simulink model "Leg_4DOF_HGO_noise"  (R2017a)
settings: Solver=FixedStepAuto  StartTime=0.0  StopTime=15  FixedStep=simulation_step  MaxStep=1e-2  RelTol=1e-3  EnableMultiTasking=on
values from neighbouring files (symbols this model uses):
  Amp = [ 1 ; pi/2*ones(3,1) ]    [Copy_of_Init_4DOF.m]
  Ar = [zeros(4) eye(4); zeros(4) zeros(4)]    [Copy_of_Init_HGO_v2.m]    (also in Init_HGO.m; Init_HGO_v1.m; Init_HGO_zoh_v2.m)
  beta = 10    [Copy_of_Init_4DOF.m]
  BodyContact = [ 4 4 ]    [Copy_of_Init_4DOF.m]
  BodyContactPositions = [ contact_point_h, contact_point_t ]    [Copy_of_Init_4DOF.m]
  Br = [zeros(4); eye(4)]    [Copy_of_Init_HGO_v2.m]    (also in Init_HGO.m; Init_HGO_v1.m; Init_HGO_zoh_v2.m)
  Cr = [eye(4) zeros(4)]    [Copy_of_Init_HGO_v2.m]    (also in Init_HGO.m; Init_HGO_v1.m; Init_HGO_zoh_v2.m)
  dqInit = [ 0 0 0 0 ]'    [Copy_of_Init_4DOF.m]
  G = g*ez    [Copy_of_Init_4DOF.m]
  G_ctrl = g*ez    [Copy_of_Init_4DOF.m]
  h = [ ez -ey -ey -ey ]    [Copy_of_Init_4DOF.m]
  h_ctrl = [ ez -ey -ey -ey ]    [Copy_of_Init_4DOF.m]
  Hmu = [eye(4)/Mu zeros(4); zeros(4) eye(4)/Mu^2]    [Copy_of_Init_HGO_v2.m]    (also in Init_HGO.m; Init_HGO_v1.m; Init_HGO_zoh_v2.m)
  Inertia = [ I_base I_hip I_thigh I_shin I_foot ]    [Copy_of_Init_4DOF.m]
  Inertia_ctrl = [ I_base I_hip I_thigh I_shin I_foot ]    [Copy_of_Init_4DOF.m]
  joint_type = [ 1 0 0 0 ]    [Copy_of_Init_4DOF.m]
  k_b = 10    [Copy_of_Init_4DOF.m]
  Kd = kd*eye(n)    [Copy_of_Init_4DOF.m]
  Ki = ki*eye(n)    [Copy_of_Init_4DOF.m]
  Kp = kp*eye(n)    [Copy_of_Init_4DOF.m]
  L = [ l_base_hip l_hip_thigh l_thigh_shin l_shin_foot ]    [Copy_of_Init_4DOF.m]
  L_ctrl = [ l_base_hip l_hip_thigh l_thigh_shin l_shin_foot ]    [Copy_of_Init_4DOF.m]
  L_hgo = [2*eye(4);6*eye(4)]    [Copy_of_Init_HGO_v2.m]    (also in Init_HGO.m = [eye(4);2*eye(4)]; Init_HGO_v1.m = [eye(4);2*eye(4)]; Init_HGO_zoh_v2.m)
  Mass = [ mass_base mass_hip mass_thigh mass_shin mass_foot ]    [Copy_of_Init_4DOF.m]
  Mass_ctrl = [ mass_base mass_hip mass_thigh mass_shin mass_foot ]    [Copy_of_Init_4DOF.m]
  Mu = 1e-3    (= 0.001)    [Copy_of_Init_HGO_v2.m]    (also in Init_HGO.m = 0.005; Init_HGO_v1.m; Init_HGO_zoh_v2.m = 1e-05)
  offset = zeros(n,1)    [Copy_of_Init_4DOF.m]
  qInit = [ 0 pi/2 -pi/2 0 ]'    [Copy_of_Init_4DOF.m]
  R = [ r_base r_hip r_thigh r_shin r_foot ]    [Copy_of_Init_4DOF.m]
  R_ctrl = [ r_base r_hip r_thigh r_shin r_foot ]    [Copy_of_Init_4DOF.m]
  s_z = 2    [Copy_of_Init_4DOF.m]
  w = [ 0   ; 0.5*pi*ones(3,1) ]    [Copy_of_Init_4DOF.m]
undefined symbols (not defined in the file or in its folder): filter_pole, Fstate0, magnitude, simulation_step, step_period
libraries: commchan3 x1
Description:
  | ------ 2018-03-01
  | ------V2
  | Versão com realimentacao de estados estimados (HGO), apresenta
  | resposta lenta devido ao pico no inicio das estimativas.
  | Ainda nao possui medidor de SNR.
settings Model: Creator=Ultron  LastModifiedBy=ignacio
settings DataIOCC: LimitDataPoints=on  SaveFormat=Array
settings OptimizationCC: LifeSpan=inf
settings DebuggingCC: SFUnexpectedBacktrackingDiag=warning  SFNoUnconditionalDefaultTransitionDiag=warning  SFExecutionAtInitializationDiag=none
settings HardwareCC: ProdBitPerPointer=32  ProdBitPerSizeT=32  ProdBitPerPtrDiffT=32  ProdLargestAtomicFloat=None  ProdIntDivRoundTo=Undefined  ProdEndianess=Unspecified  ProdWordSize=32  ProdHWDeviceType=32-bit Generic
settings ModelReferenceCC: PropagateSignalLabelsOutOfModel=off
settings GRTTargetCC: TargetLangStandard=C89/C90 (ANSI)  GeneratePreprocessorConditionals=Disable all
settings ConfigComp: CovMetricSettings=dw  CovHtmlReporting=on  CovSaveCumulativeToWorkspaceVar=on  CovSaveSingleToWorkspaceVar=on  CovExternalEMLEnable=off

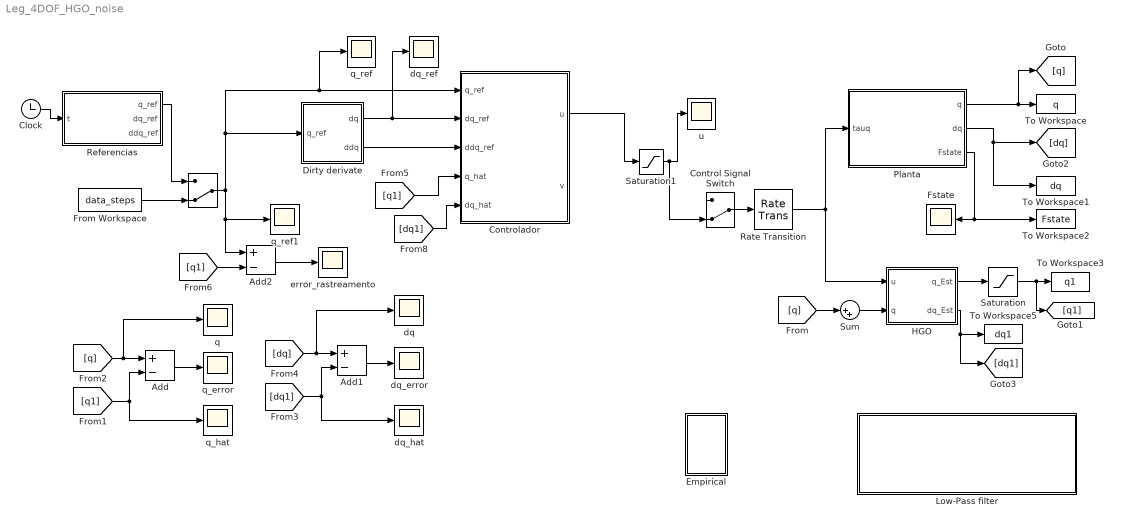
== system Leg_4DOF_HGO_noise ==
  " " : ManualSwitch  CurrentSetting=0
  Add : Sum  Inputs=+-
  Add1 : Sum  Inputs=+-
  Add2 : Sum  Inputs=+-
  Clock : Clock
  Control Signal Switch : ManualSwitch  CurrentSetting=0
  Controlador : Subsystem
  Dirty derivate : Subsystem
  Empirical : Subsystem
  From Workspace : FromWorkspace  VariableName=data_steps  SampleTime=0
  Fstate : Scope
  HGO : Subsystem
  Low-Pass filter : Subsystem
  Planta : Subsystem
  Rate Transition : RateTransition  OutPortSampleTime=simulation_step
  Referencias : MATLAB Function  TreatAsAtomicUnit=on
  Saturation : Saturate  UpperLimit=6*pi  LowerLimit=-6*pi
  Saturation1 : Saturate  UpperLimit=500  LowerLimit=-500
  Sum : Sum  Inputs=|++
  To Workspace : ToWorkspace  VariableName=q  SaveFormat=Timeseries  SampleTime=-1
  To Workspace1 : ToWorkspace  VariableName=dq  SaveFormat=Timeseries  SampleTime=-1
  To Workspace2 : ToWorkspace  VariableName=Fstate  SaveFormat=Timeseries  SampleTime=-1
  To Workspace3 : ToWorkspace  VariableName=q1  SaveFormat=Timeseries  SampleTime=-1
  To Workspace5 : ToWorkspace  VariableName=dq1  SaveFormat=Timeseries  SampleTime=-1
  dq : Scope
  dq_error : Scope
  dq_hat : Scope
  dq_ref : Scope
  error_rastreamento : Scope
  q : Scope
  q_error : Scope
  q_hat : Scope
  q_ref : Scope
  q_ref1 : Scope
  u : Scope
  wires:
  HGO/2(dq_Est) -> To Workspace5/1, [dq1]
  Sum/1 -> HGO/2(q)
  [q] -> Sum/1
  Saturation/1 -> [q1], To Workspace3/1
  [q1] -> q_hat/1, Add/2
  Clock/1 -> Referencias/1(t)
  [dq] -> dq/1, Add1/1
  Dirty derivate/2(ddq) -> Controlador/3(ddq_ref)
  Rate Transition/1 -> HGO/1(u), Planta/1(tauq)
  Dirty derivate/1(dq) -> dq_ref/1, Controlador/2(dq_ref)
  [dq1] -> dq_hat/1, Add1/2
  [q1] -> Controlador/4(q_hat)
  Planta/3(Fstate) -> Fstate/1, To Workspace2/1
  Referencias/1(q_ref) -> " "/1
  Add1/1 -> dq_error/1
  From Workspace/1 -> " "/2
  " "/1 -> Add2/1, q_ref1/1, Controlador/1(q_ref), q_ref/1, Dirty derivate/1(q_ref)
  HGO/1(q_Est) -> Saturation/1
  Planta/2(dq) -> To Workspace1/1, [dq]
  [dq1] -> Controlador/5(dq_hat)
  [q] -> q/1, Add/1
  Saturation1/1 -> Control Signal Switch/2, u/1
  Control Signal Switch/1 -> Rate Transition/1
  Controlador/1(u) -> Saturation1/1
  Add/1 -> q_error/1
  Planta/1(q) -> To Workspace/1, [q]
  [q1] -> Add2/2
  Add2/1 -> error_rastreamento/1

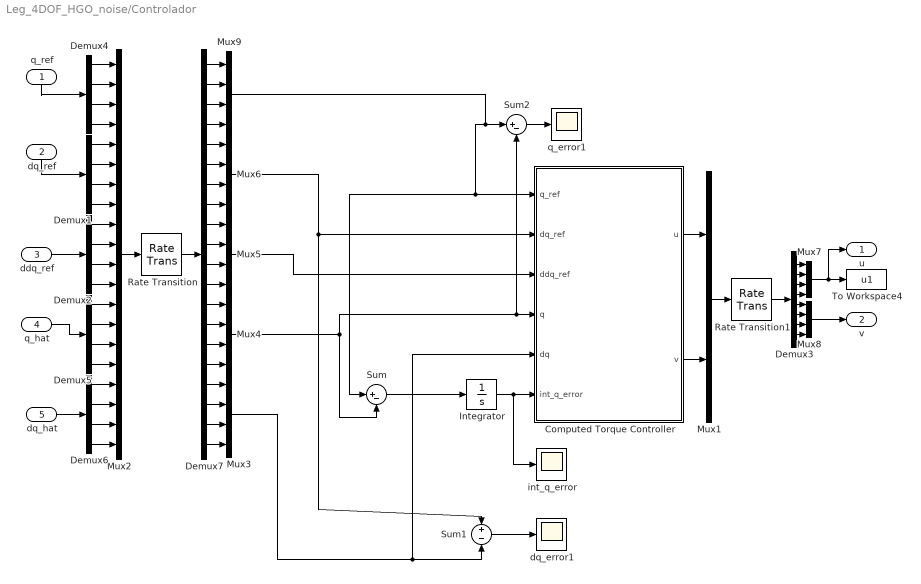
== system Leg_4DOF_HGO_noise/Controlador ==
  q_ref : Inport
  dq_ref : Inport  Port=2
  ddq_ref : Inport  Port=3
  q_hat : Inport  Port=4
  dq_hat : Inport  Port=5
  Computed Torque Controller : MATLAB Function  TreatAsAtomicUnit=on
  Demux{1..2,4..6} (5 alike) : Demux
  Demux3 : Demux  Outputs=8
  Demux7 : Demux  Outputs=20
  Integrator : Integrator  InitialCondition=zeros(4,1)
  Mux1 : Mux  Inputs=2
  Mux2 : Mux  Inputs=20
  Mux{3..9} (7 alike) : Mux
  Rate Transition : RateTransition  OutPortSampleTime=simulation_step
  Rate Transition1 : RateTransition  OutPortSampleTime=1e-3
  Sum : Sum  Inputs=|+-
  Sum1 : Sum  Inputs=+|-
  Sum2 : Sum  Inputs=|+-
  To Workspace4 : ToWorkspace  VariableName=u1  SaveFormat=Timeseries  SampleTime=-1
  dq_error1 : Scope
  int_q_error : Scope
  q_error1 : Scope
  u : Outport
  v : Outport  Port=2
  wires:
  Demux3/6 -> Mux8/2
  Demux6/3 -> Mux2/19
  Demux7/20 -> Mux3/4
  Mux3/1 -> Sum1/2, Computed Torque Controller/5(dq)
  dq_hat/1 -> Demux6/1
  Computed Torque Controller/1(u) -> Mux1/1
  Demux2/1 -> Mux2/9
  Demux1/3 -> Mux2/7
  Demux3/2 -> Mux7/2
  Sum1/1 -> dq_error1/1
  Demux6/2 -> Mux2/18
  q_ref/1 -> Demux4/1
  Demux5/4 -> Mux2/16
  Demux7/7 -> Mux6/3
  Demux7/16 -> Mux4/4
  Demux5/2 -> Mux2/14
  Demux7/3 -> Mux9/3
  Demux1/1 -> Mux2/5
  Demux6/1 -> Mux2/17
  Demux3/5 -> Mux8/1
  Mux6/1 -> Sum1/1, Computed Torque Controller/2(dq_ref)
  Demux3/4 -> Mux7/4
  q_hat/1 -> Demux5/1
  Demux7/5 -> Mux6/1
  Demux6/4 -> Mux2/20
  Demux3/3 -> Mux7/3
  Demux1/4 -> Mux2/8
  Mux9/1 -> Sum/1, Computed Torque Controller/1(q_ref), Sum2/1
  Mux8/1 -> v/1
  Mux4/1 -> Sum/2, Computed Torque Controller/4(q), Sum2/2
  Demux5/1 -> Mux2/13
  dq_ref/1 -> Demux1/1
  Demux2/3 -> Mux2/11
  Demux4/1 -> Mux2/1
  ddq_ref/1 -> Demux2/1
  Demux7/13 -> Mux4/1
  Demux3/7 -> Mux8/3
  Demux1/2 -> Mux2/6
  Demux2/4 -> Mux2/12
  Demux7/8 -> Mux6/4
  Demux7/6 -> Mux6/2
  Demux7/11 -> Mux5/3
  Demux7/9 -> Mux5/1
  Demux7/19 -> Mux3/3
  Demux7/1 -> Mux9/1
  Demux3/1 -> Mux7/1
  Sum2/1 -> q_error1/1
  Demux7/4 -> Mux9/4
  Demux7/14 -> Mux4/2
  Demux4/4 -> Mux2/4
  Demux7/12 -> Mux5/4
  Mux5/1 -> Computed Torque Controller/3(ddq_ref)
  Demux2/2 -> Mux2/10
  Demux7/2 -> Mux9/2
  Demux7/10 -> Mux5/2
  Integrator/1 -> int_q_error/1, Computed Torque Controller/6(int_q_error)
  Demux7/17 -> Mux3/1
  Demux7/18 -> Mux3/2
  Demux4/2 -> Mux2/2
  Sum/1 -> Integrator/1
  Computed Torque Controller/2(v) -> Mux1/2
  Demux3/8 -> Mux8/4
  Mux7/1 -> To Workspace4/1, u/1
  Demux4/3 -> Mux2/3
  Demux7/15 -> Mux4/3
  Demux5/3 -> Mux2/15
  Mux2/1 -> Rate Transition/1
  Rate Transition/1 -> Demux7/1
  Mux1/1 -> Rate Transition1/1
  Rate Transition1/1 -> Demux3/1

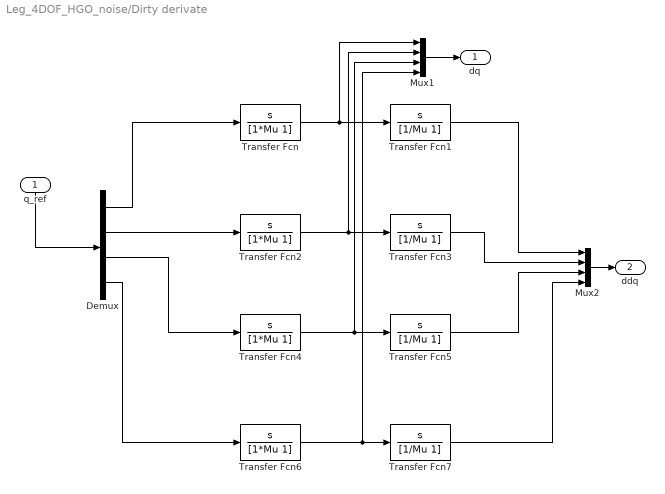
== system Leg_4DOF_HGO_noise/Dirty derivate ==
  q_ref : Inport
  Demux : Demux
  Mux1 : Mux
  Mux2 : Mux
  Transfer Fcn{,2,4,6} (4 alike) : TransferFcn  Numerator=[1 0]  Denominator=[1*Mu 1]
  Transfer Fcn{1,3,5,7} (4 alike) : TransferFcn  Numerator=[1 0]  Denominator=[1/Mu 1]
  dq : Outport
  ddq : Outport  Port=2
  wires:
  Transfer Fcn/1 -> Mux1/1, Transfer Fcn1/1
  q_ref/1 -> Demux/1
  Demux/1 -> Transfer Fcn/1
  Transfer Fcn6/1 -> Mux1/4, Transfer Fcn7/1
  Demux/2 -> Transfer Fcn2/1
  Demux/3 -> Transfer Fcn4/1
  Demux/4 -> Transfer Fcn6/1
  Mux1/1 -> dq/1
  Transfer Fcn4/1 -> Mux1/3, Transfer Fcn5/1
  Transfer Fcn2/1 -> Mux1/2, Transfer Fcn3/1
  Transfer Fcn1/1 -> Mux2/1
  Transfer Fcn3/1 -> Mux2/2
  Transfer Fcn5/1 -> Mux2/3
  Mux2/1 -> ddq/1
  Transfer Fcn7/1 -> Mux2/4

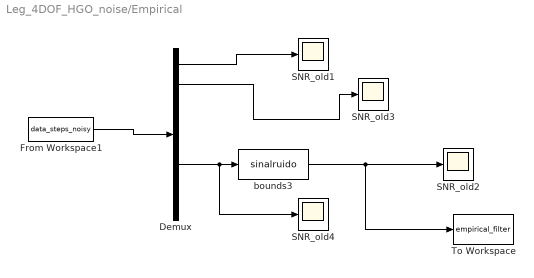
== system Leg_4DOF_HGO_noise/Empirical ==
  Demux : Demux  Outputs=8
  From Workspace1 : FromWorkspace  VariableName=data_steps_noisy  SampleTime=0
  SNR_old{1..4} (4 alike) : Scope
  To Workspace : ToWorkspace  VariableName=empirical_filter  SampleTime=-1
      settings: Save2DSignal=2-D array (concatenate along first dimension)
  bounds3 : MATLABFcn  MATLABFcn=sinalruido  Output1D=off
  wires:
  Demux/6 -> SNR_old4/1, bounds3/1
  Demux/2 -> SNR_old3/1
  Demux/1 -> SNR_old1/1
  From Workspace1/1 -> Demux/1
  bounds3/1 -> To Workspace/1, SNR_old2/1

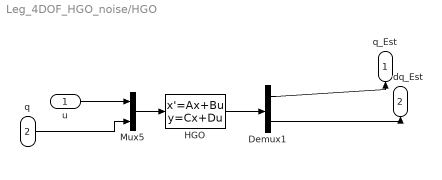
== system Leg_4DOF_HGO_noise/HGO ==
  u : Inport
  q : Inport  Port=2
  Demux1 : Demux  Outputs=2
  HGO : StateSpace  A=Ar-Hmu*L_hgo*Cr  B=[Br Hmu*L_hgo]  C=eye(8)  D=zeros(8)  X0=[0.0181; 0.5; -0.15; -0.38; 0.0; 0.0; 0.0; 0.0]
  Mux5 : Mux  Inputs=2
  q_Est : Outport  PortDimensions=4
  dq_Est : Outport  Port=2  PortDimensions=4
  wires:
  Mux5/1 -> HGO/1
  Demux1/1 -> q_Est/1
  Demux1/2 -> dq_Est/1
  u/1 -> Mux5/1
  q/1 -> Mux5/2
  HGO/1 -> Demux1/1

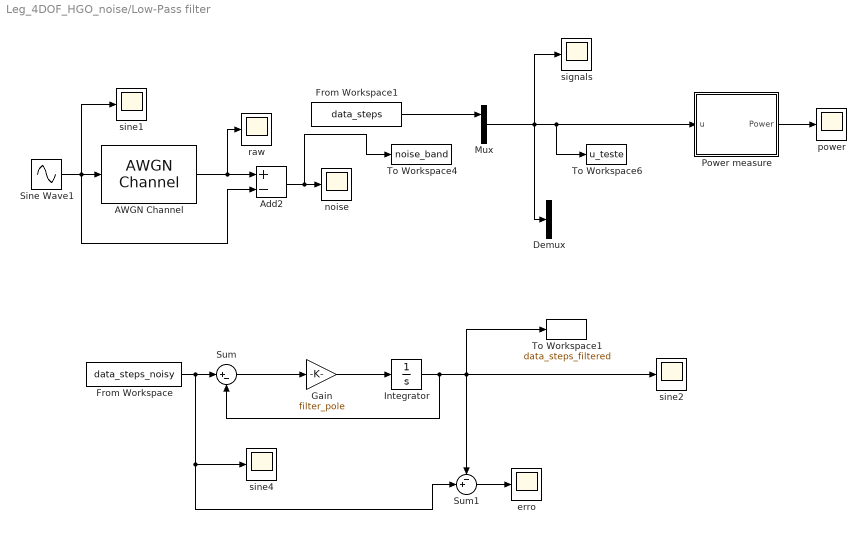
== system Leg_4DOF_HGO_noise/Low-Pass filter ==
  AWGN Channel : commchan3/AWGN Channel  InputProcessing=Columns as channels (frame based)  seed=67  noiseMode="Signal to noise ratio  (SNR)"  EbNodB=10  EsNodB=10  SNRdB=30  bitsPerSym=1  Ps=1  Tsym=1  variance=1
  Add2 : Sum  Inputs=+-
  Demux : Demux  Outputs=5
  From Workspace : FromWorkspace  VariableName=data_steps_noisy  SampleTime=0
  From Workspace1 : FromWorkspace  VariableName=data_steps  SampleTime=0
  Gain : Gain  Gain=filter_pole
  Integrator : Integrator
  Mux : Mux  Inputs=2
  Power measure : Subsystem  mask(Measure power){window=0.1, sampling=1e-3}
      mask prompts: window "Window Length"
      mask help: Foo bar
      mask init:
      | global step_period;
      | 
      | N = step_period / window;
  Sine Wave1 : Sin  Amplitude=2  Frequency=2*pi / (2 * step_period)  SampleTime=0
  Sum : Sum  Inputs=|+-
  Sum1 : Sum  Inputs=-+|
  To Workspace1 : ToWorkspace  VariableName=data_steps_filtered  SaveFormat=Timeseries  SampleTime=-1
  To Workspace4 : ToWorkspace  VariableName=noise_band  SaveFormat=Timeseries  SampleTime=-1
  To Workspace6 : ToWorkspace  VariableName=u_teste  SaveFormat=Timeseries  SampleTime=-1
  erro : Scope
  noise : Scope
  power : Scope
  raw : Scope
  signals : Scope
  sine1 : Scope
  sine2 : Scope
  sine4 : Scope
  wires:
  Mux/1 -> Demux/1, To Workspace6/1, Power measure/1(u), signals/1
  Add2/1 -> To Workspace4/1, noise/1
  AWGN Channel/1 -> raw/1, Add2/1
  Power measure/1(Power) -> power/1
  From Workspace1/1 -> Mux/1
  Sine Wave1/1 -> Add2/2, sine1/1, AWGN Channel/1
  Gain/1 -> Integrator/1
  Sum/1 -> Gain/1
  From Workspace/1 -> Sum1/2, sine4/1, Sum/1
  Integrator/1 -> To Workspace1/1, sine2/1, Sum1/1, Sum/2
  Sum1/1 -> erro/1

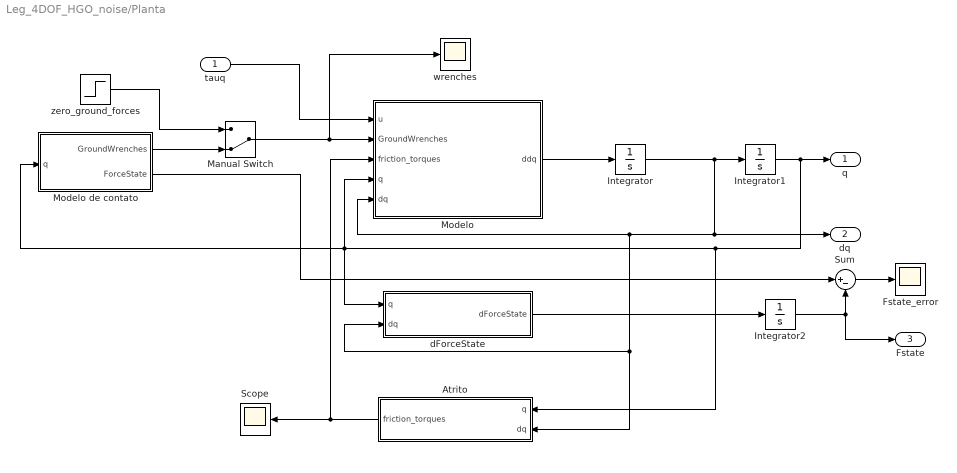
== system Leg_4DOF_HGO_noise/Planta ==
  tauq : Inport
  Atrito : MATLAB Function  TreatAsAtomicUnit=on
  Fstate_error : Scope
  Integrator : Integrator  InitialCondition=dqInit
  Integrator1 : Integrator  InitialCondition=qInit
  Integrator2 : Integrator  InitialCondition=Fstate0
  Manual Switch : ManualSwitch  CurrentSetting=0
  Modelo : MATLAB Function  TreatAsAtomicUnit=on
  Modelo de contato : MATLAB Function  TreatAsAtomicUnit=on
  Scope : Scope
  Sum : Sum  Inputs=|+-
  dForceState : MATLAB Function  TreatAsAtomicUnit=on
  wrenches : Scope
  zero_ground_forces : Step  Before=zeros(6,2)  After=zeros(6,2)  SampleTime=simulation_step
  q : Outport
  dq : Outport  Port=2
  Fstate : Outport  Port=3
  wires:
  Integrator1/1 -> dForceState/1(q), Modelo de contato/1(q), Modelo/4(q), Atrito/1(q), q/1
  Integrator/1 -> Integrator1/1, Modelo/5(dq), dForceState/2(dq), Atrito/2(dq), dq/1
  Atrito/1(friction_torques) -> Modelo/3(friction_torques), Scope/1
  tauq/1 -> Modelo/1(u)
  Integrator2/1 -> Sum/2, Fstate/1
  dForceState/1(dForceState) -> Integrator2/1
  Modelo de contato/2(ForceState) -> Sum/1
  Sum/1 -> Fstate_error/1
  Manual Switch/1 -> wrenches/1, Modelo/2(GroundWrenches)
  Modelo de contato/1(GroundWrenches) -> Manual Switch/2
  zero_ground_forces/1 -> Manual Switch/1
  Modelo/1(ddq) -> Integrator/1

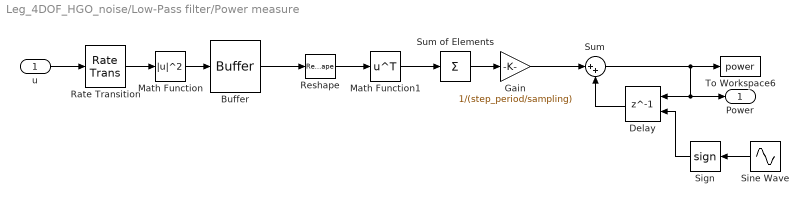
== system Leg_4DOF_HGO_noise/Low-Pass filter/Power measure ==
  u : Inport
  Buffer : Buffer  N=5 * window/sampling  OutputFrames=off
  Delay : Delay  DelayLength=1  ExternalReset=Either
      settings: InputPortMap=u0,r5
  Gain : Gain  Gain=1/(step_period/sampling)
  Math Function : Math  Operator=magnitude^2  SaturateOnIntegerOverflow=on
  Math Function1 : Math  Operator=transpose  SaturateOnIntegerOverflow=on
  Rate Transition : RateTransition  OutPortSampleTime=sampling
  Reshape : Reshape  OutputDimensionality=Customize  OutputDimensions=[5,window/sampling]
  Sign : Signum
  Sine Wave : Sin  Frequency=2*pi / (2 * step_period)  SampleTime=window
  Sum : Sum  Inputs=|++
  Sum of Elements : Sum  Inputs=+  CollapseMode=Specified dimension
  To Workspace6 : ToWorkspace  VariableName=power  SaveFormat=Timeseries  SampleTime=-1
  Power : Outport
  wires:
  Math Function/1 -> Buffer/1
  Rate Transition/1 -> Math Function/1
  Gain/1 -> Sum/1
  Reshape/1 -> Math Function1/1
  Sum of Elements/1 -> Gain/1
  Buffer/1 -> Reshape/1
  Math Function1/1 -> Sum of Elements/1
  Sum/1 -> Delay/1, Power/1, To Workspace6/1
  Delay/1 -> Sum/2
  Sine Wave/1 -> Sign/1
  Sign/1 -> Delay/2
  u/1 -> Rate Transition/1

== matlab function Leg_4DOF_HGO_noise/Planta/Modelo ==
  data: u input; GroundWrenches input; friction_torques input; q input; dq input; joint_type parameter; Mass parameter; Inertia parameter; R parameter; L parameter; h parameter; G parameter; ddq output; BodyContactPositions parameter; BodyContact parameter
function ddq = fcn( u, GroundWrenches, friction_torques, q, dq, joint_type, Mass, Inertia, R, L, h, G, BodyContactPositions,  BodyContact )
% direct dynamics

% n = length(q);

% coder.extrinsic('model_prosthetics_mex');
% ddq = coder.nullcopy(zeros(n,1));
% Friction_torques = coder.nullcopy(zeros(n,1));

ddq = model_prosthetics( u, q, dq, joint_type, Mass, Inertia, R, L, h, G, friction_torques, BodyContact, GroundWrenches, BodyContactPositions );
% ddq = model_prosthetics_mex( u, q, dq, joint_type, Mass, Inertia, R, L, h, G, friction_coefs, BodyContact, BodyContactWrenches, BodyContactPositions );

== matlab function Leg_4DOF_HGO_noise/Referencias ==
  data: t input; q_ref output; Amp parameter; offset parameter; w parameter; dq_ref output; ddq_ref output
function [q_ref, dq_ref, ddq_ref] = fcn( t, Amp, offset, w)
% generate reference

% q_ref = A*sin(w*t + offset);
% dq_ref = A*w*cos(w*t + offset);
% ddq_ref = -A*(w^2)*sin(w*t + offset);

q_ref = zeros(4,1);
dq_ref = zeros(4,1);
ddq_ref = zeros(4,1);

for i = 1:4
    q_ref(i) = Amp(i)*sin(w(i)*t + offset(i));
    dq_ref(i) = Amp(i)*w(i)*cos(w(i)*t + offset(i));
    ddq_ref(i) = -Amp(i)*(w(i)^2)*sin(w(i)*t + offset(i));
end

== matlab function Leg_4DOF_HGO_noise/Planta/Atrito ==
  data: friction_torques output; q input; dq input
function friction_torques = fcn( q, dq )
%% Joint friction model
n = length(q);
friction_torques = zeros(n,1);

== matlab function Leg_4DOF_HGO_noise/Controlador/Computed Torque Controller ==
  data: q_ref input; dq_ref input; ddq_ref input; u output; q input; dq input; int_q_error input; joint_type parameter; Mass_ctrl parameter; Inertia_ctrl parameter; R_ctrl parameter; L_ctrl parameter; h_ctrl parameter; G_ctrl parameter; Kp parameter; Kd parameter; Ki parameter; v output
function [u,v] = fcn(q_ref, dq_ref, ddq_ref, q, dq, int_q_error, joint_type, Mass_ctrl, Inertia_ctrl, R_ctrl, L_ctrl, h_ctrl, G_ctrl, Kp, Kd, Ki )
%% Prostectics control

v = ddq_ref + Kd*(dq_ref - dq) + Kp*(q_ref - q) + Ki*int_q_error;
u = prosthetics_inverse_dynamics( q, dq, v, joint_type, Mass_ctrl, Inertia_ctrl, R_ctrl, L_ctrl, h_ctrl, G_ctrl );

== matlab function Leg_4DOF_HGO_noise/Planta/Modelo de contato ==
  data: GroundWrenches output; q input; BodyContactPositions parameter; s_z parameter; L parameter; h parameter; beta parameter; k_b parameter; joint_type parameter; ForceState output
function [ GroundWrenches, ForceState ] = fcn( q, BodyContactPositions, s_z, L, h, beta,  k_b, joint_type )
% function BodyContactWrenches = fcn( t, q, L, h, BodyContactPositions, joint_type, sz, beta, kb)
% Esta função calcula as forças de contato com o chão

[ GroundWrenches, ForceState ] = ground_model( q, BodyContactPositions, s_z, L, h, beta,  k_b, joint_type );

== matlab function Leg_4DOF_HGO_noise/Planta/dForceState ==
  data: q input; dq input; dForceState output; L parameter; h parameter; joint_type parameter; BodyContactPositions parameter; s_z parameter; beta parameter; k_b parameter
function dForceState = fcn( q, dq, L, h, joint_type,  BodyContactPositions, s_z, beta, k_b)
%% Dinâmica do modelo de contato (em coordenadas inerciais)

%% Computes the velocity body twist of the given point.
body = 4;
contact_point_h = BodyContactPositions(:,1);
contact_point_t = BodyContactPositions(:,2);
V_h = prosthetics_diff_kinematics( q, dq, L, h, body, contact_point_h, joint_type );
V_t = prosthetics_diff_kinematics( q, dq, L, h, body, contact_point_t, joint_type );

%% Computes 
[ P_h, R_h ] = prosthetics_forward_kinematics( q, L, h, body, contact_point_h, joint_type );
[ P_t, R_t ] = prosthetics_forward_kinematics( q, L, h, body, contact_point_h, joint_type );
z_h = P_h(3);
z_t = P_t(3);

%% Converts body linear velocity into inertial velocty
v_h = R_h*V_h(1:3);
v_t = R_t*V_t(1:3);

dz_h = v_h(3);
dz_t = v_t(3);

dF_zh = -(k_b/2)*dz_h*(1+sign(z_h - s_z));
dF_zt = -(k_b/2)*dz_t*(1+sign(z_t - s_z));

dF_xh = beta*dF_zh;
dF_xt = beta*dF_zt;

dForceState = [ dF_zh dF_zt dF_xh dF_xt ]';
